simulink model "model_sad"  (R2023a)
settings: Solver=VariableStepAuto  StartTime=0.0  StopTime=10.0  RelTol=1e-3
settings Model: Creator=Theomur  LastModifiedBy=Theomur

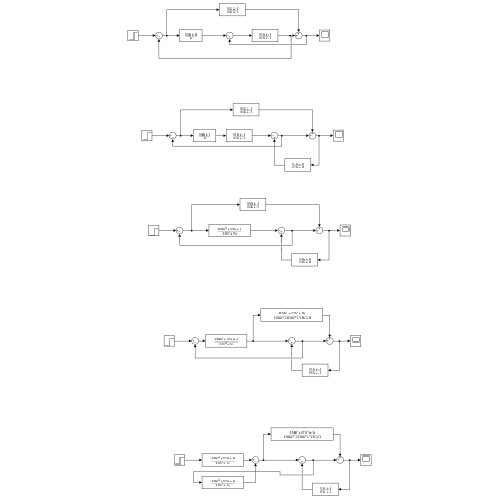
[thumbnail: Simulink's stored preview of the top-level diagram]
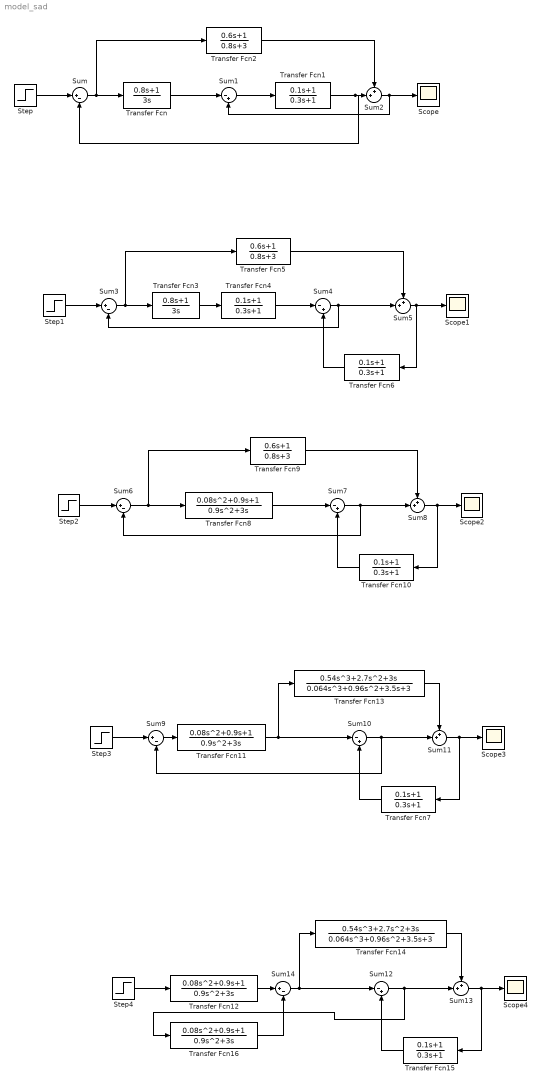
== system model_sad ==
  Scope{,1..4} (5 alike) : Scope
  Step{,1..4} (5 alike) : Step  SampleTime=0
  Sum{,3,6,9,14} (5 alike) : Sum  Inputs=|+-
  Sum{1,4,7,10,12} (5 alike) : Sum  Inputs=|-+
  Sum{2,5,8,11,13} (5 alike) : Sum  Inputs=++|
  Transfer Fcn : TransferFcn  Numerator=[0.8 1]  Denominator=[3 0]
  Transfer Fcn{1,4,6..7,10,15} (6 alike) : TransferFcn  Numerator=[0.1 1]  Denominator=[0.3 1]
  Transfer Fcn{8,11..12,16} (4 alike) : TransferFcn  Numerator=[0.08 0.9 1]  Denominator=[0.9 3 0]
  Transfer Fcn13 : TransferFcn  Numerator=[0.54 2.7 3 0]  Denominator=[0.064 0.96 3.5 3]
  Transfer Fcn14 : TransferFcn  Numerator=[0.54 2.7 3 0]  Denominator=[0.064 0.96 3.5 3]
  Transfer Fcn2 : TransferFcn  Numerator=[0.6 1]  Denominator=[0.8 3]
  Transfer Fcn3 : TransferFcn  Numerator=[0.8 1]  Denominator=[3 0]
  Transfer Fcn5 : TransferFcn  Numerator=[0.6 1]  Denominator=[0.8 3]
  Transfer Fcn9 : TransferFcn  Numerator=[0.6 1]  Denominator=[0.8 3]
  wires:
  Step/1 -> Sum/1
  Sum/1 -> Transfer Fcn2/1, Transfer Fcn/1
  Transfer Fcn/1 -> Sum1/1
  Sum1/1 -> Transfer Fcn1/1
  Transfer Fcn1/1 -> Sum/2, Sum2/2
  Sum2/1 -> Sum1/2, Scope/1
  Transfer Fcn2/1 -> Sum2/1
  Transfer Fcn5/1 -> Sum5/1
  Step1/1 -> Sum3/1
  Sum3/1 -> Transfer Fcn5/1, Transfer Fcn3/1
  Sum5/1 -> Transfer Fcn6/1, Scope1/1
  Transfer Fcn3/1 -> Transfer Fcn4/1
  Transfer Fcn4/1 -> Sum4/1
  Sum4/1 -> Sum3/2, Sum5/2
  Transfer Fcn6/1 -> Sum4/2
  Transfer Fcn10/1 -> Sum7/2
  Sum8/1 -> Transfer Fcn10/1, Scope2/1
  Transfer Fcn9/1 -> Sum8/1
  Step2/1 -> Sum6/1
  Sum6/1 -> Transfer Fcn9/1, Transfer Fcn8/1
  Sum7/1 -> Sum6/2, Sum8/2
  Transfer Fcn8/1 -> Sum7/1
  Step3/1 -> Sum9/1
  Transfer Fcn7/1 -> Sum10/2
  Sum10/1 -> Sum9/2, Sum11/2
  Sum11/1 -> Transfer Fcn7/1, Scope3/1
  Transfer Fcn13/1 -> Sum11/1
  Sum9/1 -> Transfer Fcn11/1
  Transfer Fcn11/1 -> Sum10/1, Transfer Fcn13/1
  Sum14/1 -> Transfer Fcn14/1, Sum12/1
  Transfer Fcn14/1 -> Sum13/1
  Sum12/1 -> Transfer Fcn16/1, Sum13/2
  Transfer Fcn15/1 -> Sum12/2
  Sum13/1 -> Transfer Fcn15/1, Scope4/1
  Step4/1 -> Transfer Fcn12/1
  Transfer Fcn12/1 -> Sum14/1
  Transfer Fcn16/1 -> Sum14/2
